simulink subsystem "LadderUnitLPF"  (R2024a)
settings: Solver=VariableStepAuto  StartTime=0.0  StopTime=10.0  RelTol=1e-3
settings Model: Creator=dfurodet  LastModifiedBy=dfurodet

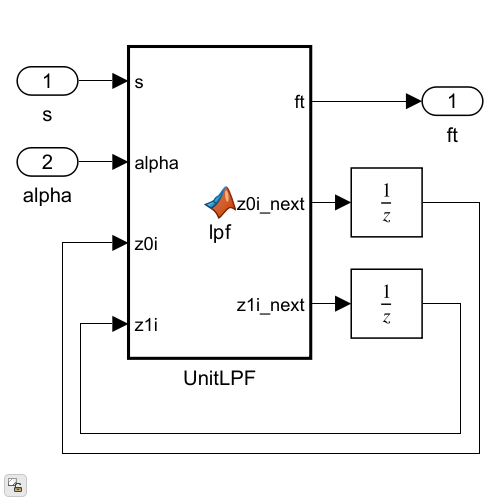
[thumbnail: Simulink's stored preview of the top-level diagram]
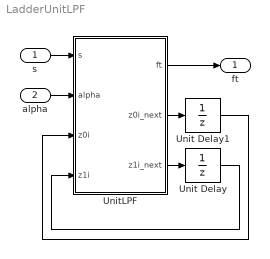
== system LadderUnitLPF ==
  s : Inport
  alpha : Inport  Port=2
  Unit Delay : UnitDelay  SampleTime=-1  HasFrameUpgradeWarning=on
  Unit Delay1 : UnitDelay  SampleTime=-1  HasFrameUpgradeWarning=on
  UnitLPF : MATLAB Function  TreatAsAtomicUnit=on
  ft : Outport
  wires:
  UnitLPF/2(z0i_next) -> Unit Delay1/1
  Unit Delay/1 -> UnitLPF/4(z1i)
  Unit Delay1/1 -> UnitLPF/3(z0i)
  s/1 -> UnitLPF/1(s)
  UnitLPF/1(ft) -> ft/1
  alpha/1 -> UnitLPF/2(alpha)
  UnitLPF/3(z1i_next) -> Unit Delay/1

== matlab function LadderUnitLPF/UnitLPF ==
  data: s input; ft output; alpha input; z0i input; z1i input; z0i_next output; z1i_next output
function [ft, z0i_next, z1i_next] = lpf(s, alpha, z0i, z1i)
ft = s * 0.76923077 + 0.23076923 * z0i - z1i;
ft = ft * alpha + z1i;
z1i_next = ft;
z0i_next = s;
